simulink model "P4E2OAAA"  (R2018a)
settings: Solver=FixedStepAuto  StartTime=0.0  StopTime=10  FixedStep=0.1  RelTol=1e-3
settings Model: Creator=Oscar  LastModifiedBy=Oscar

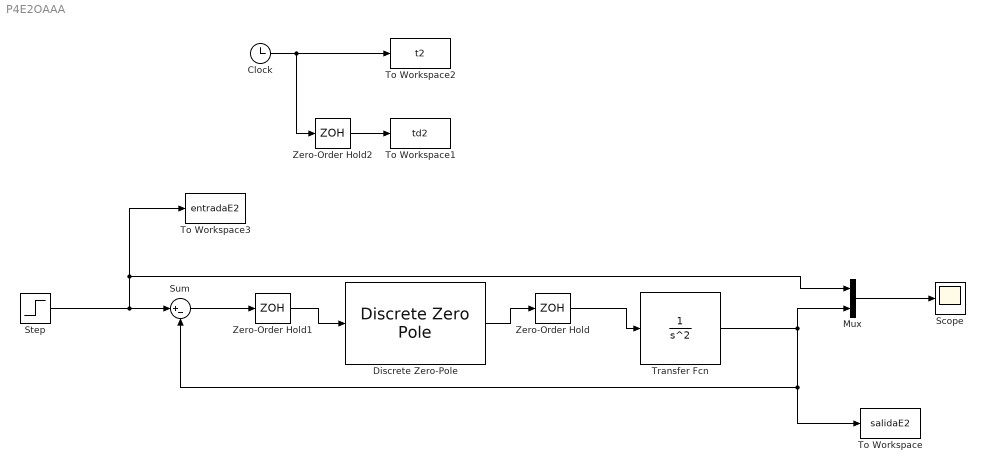
== system P4E2OAAA ==
  Clock : Clock
  Discrete Zero-Pole : DiscreteZeroPole  Zeros=[0.771]  Poles=[0]  Gain=42.71  SampleTime=0.1
  Mux : Mux  Inputs=2
  Scope : Scope
  Step : Step  Time=0  SampleTime=0.1
  Sum : Sum  Inputs=|+-
  To Workspace : ToWorkspace  VariableName=salidaE2  SampleTime=-1
  To Workspace1 : ToWorkspace  VariableName=td2  SampleTime=-1
  To Workspace2 : ToWorkspace  VariableName=t2  SampleTime=-1
  To Workspace3 : ToWorkspace  VariableName=entradaE2  SampleTime=-1
  Transfer Fcn : TransferFcn  Denominator=[1 0 0]
  Zero-Order Hold : ZeroOrderHold  SampleTime=0.1
  Zero-Order Hold1 : ZeroOrderHold  SampleTime=0.1
  Zero-Order Hold2 : ZeroOrderHold  SampleTime=0.1
  wires:
  Transfer Fcn/1 -> Mux/2, Sum/2, To Workspace/1
  Discrete Zero-Pole/1 -> Zero-Order Hold/1
  Zero-Order Hold/1 -> Transfer Fcn/1
  Step/1 -> To Workspace3/1, Mux/1, Sum/1
  Mux/1 -> Scope/1
  Clock/1 -> Zero-Order Hold2/1, To Workspace2/1
  Zero-Order Hold2/1 -> To Workspace1/1
  Zero-Order Hold1/1 -> Discrete Zero-Pole/1
  Sum/1 -> Zero-Order Hold1/1
